simulink model "ObjectTrackingMove2"  (R2020b)
settings: Solver=FixedStepAuto  StartTime=0.0  StopTime=inf  RelTol=1e-3  EnableMultiTasking=on
undefined symbols (not defined in the file or in its folder): DiscIntNeverNeededParam
libraries: embdlinuxlib x6, raspberrypiAVlib x1, raspberrypiBasiclib x1
settings Model: SimulationMode=external  Creator=wojna  LastModifiedBy=JaaW
settings SolverCC: PositivePriorityOrder=on
settings OptimizationCC: EnhancedBackFolding=on  PassReuseOutputArgsThreshold=0  MaxStackSize=64  OptimizeBlockOrder=speed  DifferentSizesBufferReuse=on  OptimizationCustomize=off
settings DebuggingCC: ParameterTunabilityLossMsg=error
settings HardwareCC: ProdBitPerPointer=32  ProdBitPerSizeT=32  ProdBitPerPtrDiffT=32  ProdLargestAtomicInteger=Long  ProdLargestAtomicFloat=Double  ProdWordSize=32  ProdLongLongMode=on  ProdHWDeviceType=ARM Compatible->ARM Cortex  UseEmbeddedCoderFeatures=off  UseSimulinkCoderFeatures=off
settings SFSimCC: MATLABDynamicMemAlloc=off  CustomCodeUndefinedFunction=UseInterfaceOnly
settings RTWCC: Description=Embedded Coder  SystemTargetFile=ert.tlc  HardwareBoard=Raspberry Pi  TLCOptions="-aInlineSetEventsForThisBaseRateFcn=TLC_FALSE -aSuppressMultiTaskScheduler=TLC_FALSE  -aRateBasedStepFcn=0"  TemplateMakefile=ert_default_tmf  GenerateReport=on  Toolchain=GNU GCC Raspberry Pi  BuildConfiguration=Faster Runs  LaunchReport=on
settings CodeAppCC: ForceParamTrailComments=on  OperatorAnnotations=on  MangleLength=10
settings ERTTargetCC: ERTCustomFileBanners=off  SupportContinuousTime=on  SupportNonInlinedSFcns=on  RemoveResetFunc=off  SupportVariableSizeSignals=on  ModelStepFunctionPrototypeControlCompliant=off

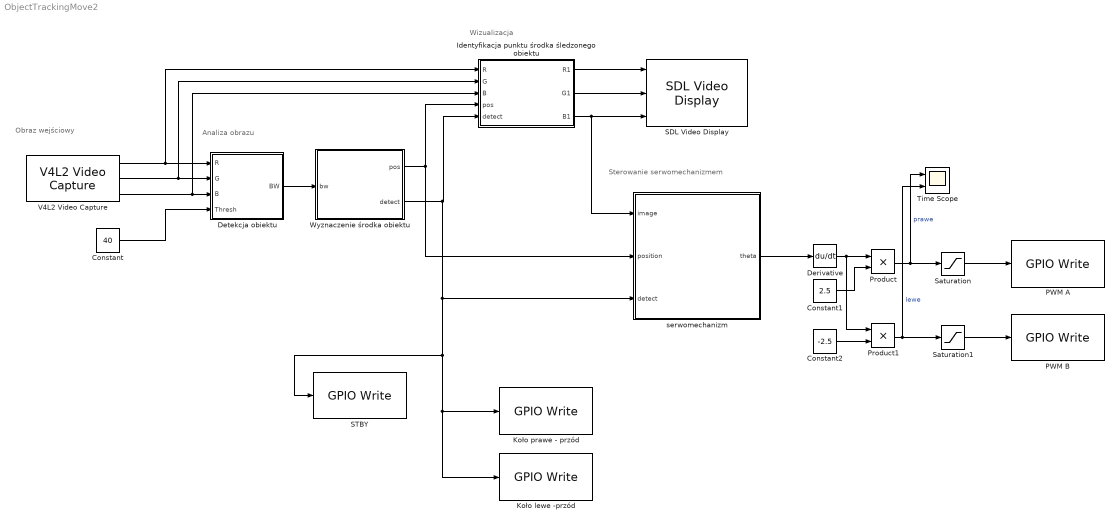
== system ObjectTrackingMove2 ==
  note: Obraz wejściowy
  note: Sterowanie serwomechanizmem
  note: Wizualizacja
  note: Analiza obrazu
  Constant : Constant  Value=40
  Constant1 : Constant  Value=2.5
  Constant2 : Constant  Value=-2.5
  Derivative : Derivative
  Detekcja obiektu : Subsystem
  Identyfikacja punktu środka śledzonego obiektu : MATLAB Function  TreatAsAtomicUnit=on
  Koło lewe -przód : embdlinuxlib/GPIO Write  board=Pi 3 Model B+  gpio=18  direction=Output  blockPlatform=Raspberry Pi
      settings: SourceProductBaseCode=SC_BEAGLEBONE_BLUE,NVIDIA,RASPPI
  Koło prawe - przód : embdlinuxlib/GPIO Write  board=Pi 3 Model B+  gpio=22  direction=Output  blockPlatform=Raspberry Pi
      settings: SourceProductBaseCode=SC_BEAGLEBONE_BLUE,NVIDIA,RASPPI
  PWM A : embdlinuxlib/GPIO Write  board=Pi 3 Model B+  gpio=20  direction=Output  blockPlatform=Raspberry Pi
      settings: SourceProductBaseCode=SC_BEAGLEBONE_BLUE,NVIDIA,RASPPI
  PWM B : embdlinuxlib/GPIO Write  board=Pi 3 Model B+  gpio=16  direction=Output  blockPlatform=Raspberry Pi
      settings: SourceProductBaseCode=SC_BEAGLEBONE_BLUE,NVIDIA,RASPPI
  Product : Product  OutMin=[0]  OutMax=[1]
  Product1 : Product  OutMin=[0]  OutMax=[1]
  SDL Video Display : embdlinuxlib/SDL Video Display  pixelFormat=RGB  pixelOrder=Planar  rowMajor=on  blockPlatform=Raspberry Pi
      settings: SourceProductBaseCode=SC_BEAGLEBONE_BLUE,NVIDIA,RASPPI
  STBY : embdlinuxlib/GPIO Write  board=Pi 3 Model B+  gpio=21  direction=Output  blockPlatform=Raspberry Pi
      settings: SourceProductBaseCode=SC_BEAGLEBONE_BLUE,NVIDIA,RASPPI
  Saturation : Saturate  LowerLimit=0
  Saturation1 : Saturate  UpperLimit=5  LowerLimit=0
  Time Scope : Scope  NumInputPorts=2
  V4L2 Video Capture : raspberrypiAVlib/V4L2 Video Capture  DeviceName=/dev/video0  Resolution=320x240  CustomResolution=[ 320, 240 ]  PixelFormat=RGB  SampleTime=0.01  pixelOrder=Planar  simOutput=Colorbars  imSizeSelection=160x120  imSize=[640, 480]  roi=[0, 0, 640, 480]  m_devName='/dev/video0'  blockPlatform=Raspberry Pi
      settings: SourceProductBaseCode=RASPPI
  Wyznaczenie środka obiektu : MATLAB Function  TreatAsAtomicUnit=on
  serwomechanizm : Subsystem
  wires:
  V4L2 Video Capture/1 -> Detekcja obiektu/1(R), Identyfikacja punktu środka śledzonego obiektu/1(R)
  V4L2 Video Capture/2 -> Detekcja obiektu/2(G), Identyfikacja punktu środka śledzonego obiektu/2(G)
  V4L2 Video Capture/3 -> Identyfikacja punktu środka śledzonego obiektu/3(B), Detekcja obiektu/3(B)
  Detekcja obiektu/1(BW) -> Wyznaczenie środka obiektu/1(bw)
  Wyznaczenie środka obiektu/1(pos) -> Identyfikacja punktu środka śledzonego obiektu/4(pos), serwomechanizm/2(position)
  Wyznaczenie środka obiektu/2(detect) -> STBY/1, Koło lewe -przód/1, Koło prawe - przód/1, serwomechanizm/3(detect), Identyfikacja punktu środka śledzonego obiektu/5(detect)
  Identyfikacja punktu środka śledzonego obiektu/1(R1) -> SDL Video Display/1
  Identyfikacja punktu środka śledzonego obiektu/2(G1) -> SDL Video Display/2
  Identyfikacja punktu środka śledzonego obiektu/3(B1) -> serwomechanizm/1(image), SDL Video Display/3
  Constant/1 -> Detekcja obiektu/4(Thresh)
  Derivative/1 -> Product/1, Product1/1
  Constant1/1 -> Product/2
  Constant2/1 -> Product1/2
  Product/1 -> Saturation/1, Time Scope/1  "prawe"
  Product1/1 -> Saturation1/1, Time Scope/2  "lewe"
  Saturation1/1 -> PWM B/1
  Saturation/1 -> PWM A/1
  serwomechanizm/1(theta) -> Derivative/1

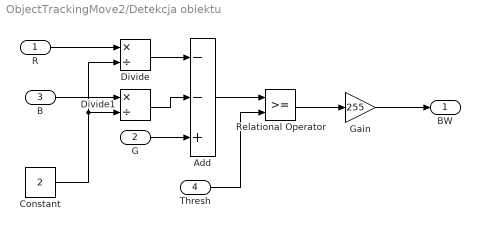
== system ObjectTrackingMove2/Detekcja obiektu ==
  R : Inport
  G : Inport  Port=2
  B : Inport  Port=3
  Thresh : Inport  Port=4
  Add : Sum  Inputs=--+
  Constant : Constant  Value=2
  Divide : Product  Inputs=*/
  Divide1 : Product  Inputs=*/
  Gain : Gain  Gain=255
  Relational Operator : RelationalOperator  OutDataTypeStr=boolean  RndMeth=Simplest
  BW : Outport  VectorParamsAs1DForOutWhenUnconnected=off
  wires:
  Thresh/1 -> Relational Operator/2
  Constant/1 -> Divide1/2, Divide/2
  Gain/1 -> BW/1
  Add/1 -> Relational Operator/1
  Divide1/1 -> Add/2
  Relational Operator/1 -> Gain/1
  Divide/1 -> Add/1
  R/1 -> Divide/1
  B/1 -> Divide1/1
  G/1 -> Add/3

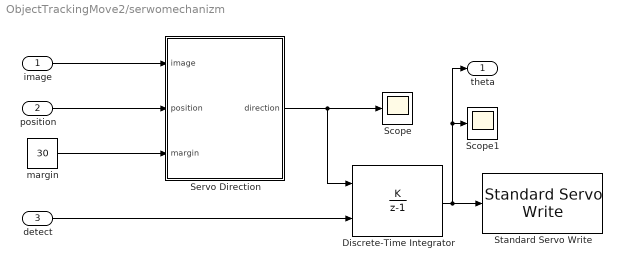
== system ObjectTrackingMove2/serwomechanizm ==
  image : Inport
  position : Inport  Port=2
  detect : Inport  Port=3
  Discrete-Time Integrator : DiscreteIntegrator  IntegratorMethod=Accumulation: Forward Euler  ExternalReset=falling  InitialCondition=90  SampleTime=-1  LimitOutput=on  UpperSaturationLimit=180  LowerSaturationLimit=0  ICPrevOutput=DiscIntNeverNeededParam  ICPrevScaledInput=DiscIntNeverNeededParam
  Scope : Scope
  Scope1 : Scope
  "Servo Direction " : Subsystem
  Standard Servo Write : raspberrypiBasiclib/Standard Servo Write  board=Pi 3 Model B  Pin_=26  MinPulseDuration=1000e-6  MaxPulseDuration=2000e-6  blockPlatform=Raspberry Pi
      settings: SourceProductBaseCode=RASPPI
  margin : Constant  Value=30
  theta : Outport  VectorParamsAs1DForOutWhenUnconnected=off
  wires:
  "Servo Direction "/1("direction ") -> Discrete-Time Integrator/1, Scope/1
  detect/1 -> Discrete-Time Integrator/2
  Discrete-Time Integrator/1 -> Standard Servo Write/1, theta/1, Scope1/1
  margin/1 -> "Servo Direction "/3("margin ")
  position/1 -> "Servo Direction "/2(position)
  image/1 -> "Servo Direction "/1(image)

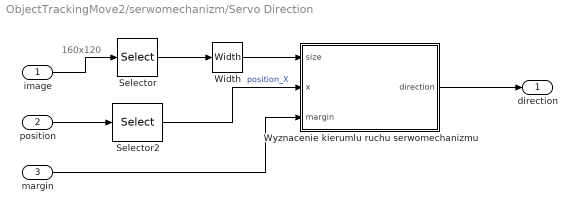
== system ObjectTrackingMove2/serwomechanizm/Servo Direction  ==
  note: 160x120
  image : Inport
  position : Inport  Port=2
  "margin " : Inport  Port=3
  Selector : Selector  NumberOfDimensions=2  InputPortWidth=160  IndexOptions=Select all,Starting index (dialog)  Indices=1,1  OutputSizes=160,1
  Selector2 : Selector  InputPortWidth=2  IndexOptions=Index vector (dialog)  Indices=1  OutputSizes=1
  Width : Width
  Wyznacenie kierumlu ruchu serwomechanizmu : MATLAB Function  TreatAsAtomicUnit=on
  "direction " : Outport  VectorParamsAs1DForOutWhenUnconnected=off
  wires:
  position/1 -> Selector2/1
  Wyznacenie kierumlu ruchu serwomechanizmu/1(direction) -> "direction "/1
  Selector2/1 -> Wyznacenie kierumlu ruchu serwomechanizmu/2(x)  "position_X"
  Width/1 -> Wyznacenie kierumlu ruchu serwomechanizmu/1(size)
  Selector/1 -> Width/1
  image/1 -> Selector/1
  "margin "/1 -> Wyznacenie kierumlu ruchu serwomechanizmu/3(margin)

== matlab function ObjectTrackingMove2/Wyznaczenie środka obiektu ==
  data: bw input; pos output; detect output
function [pos, detect] = FindCentroid(bw)

[r,c]=find(bw);
if isempty(r)
    pos = [-1 -1];
    detect = false;
else
    pos = [mean(r), mean(c)];
    detect = true;
end

== matlab function ObjectTrackingMove2/Identyfikacja punktu środka śledzonego obiektu ==
  data: R input; R1 output; G input; B input; pos input; detect input; G1 output; B1 output
function [R1,G1,B1] = MarkImage(R,G,B, pos, detect)
R1 = R; G1 = G; B1 = B;
if detect
    R1(pos(1)-3:pos(1)+3, pos(2)-3:pos(2)+3) = 255;
    G1(pos(1)-3:pos(1)+3, pos(2)-3:pos(2)+3) = 0; 
    B1(pos(1)-3:pos(1)+3, pos(2)-3:pos(2)+3) = 0;
end

== matlab function ObjectTrackingMove2/serwomechanizm/Servo Direction /Wyznacenie kierumlu ruchu serwomechanizmu ==
  data: size input; direction output; x input; margin input
function direction = servoDirection(size, x, margin)

center = size/2;
if x == -1
    direction = 0;
elseif x >= center + margin
    direction = -1;
elseif x <= center - margin
    direction = 1;
else 
    direction = 0;
end
